simulink model "inv_rot_pen_sldrt_uart_com"  (R2024a)
settings: Solver=ode3  StartTime=0.0  StopTime=inf  FixedStep=Ts  RelTol=1e-3
PostLoadFcn:
  | try
  | if isempty(which('ZHAWcbfcn'));
  | callback_fid07124=fopen('ZHAWcbfcn.m','w');
  | [~]=fprintf(callback_fid07124,'%s',get_param([bdroot,'/ Setup SLDRT'],'ClipboardFcn'));
  | [~]=fclose(callback_fid07124);
  | setpref('ZHAW_SLDRT_lib','cb_fcn',which('ZHAWcbfcn'))
  | clear callback_fid07124
  | end
  | catch
  | clear callback_fid07124
  | end
  | Ts=eval(get_param([bdroot,'/ Setup SLDRT'],'Ts'));
InitFcn:
  | Ts=eval(get_param([bdroot,'/ Setup SLDRT'],'Ts'));
values from neighbouring files (symbols this model uses):
  i_max = 0.5    [inv_rot_pen_ini.m]    (also in swing_up_inv_rot_pen_ini.m)
  phi2_disable = 10 * pi/180    (= 0.174532925199)    [inv_rot_pen_ini.m]
  phi2_enable = 30 * pi/180    (= 0.523598775598)    [inv_rot_pen_ini.m]
  V = 1 / dc(1)    [inv_rot_pen_ini.m]
undefined symbols (not defined in the file or in its folder): K, Serial_Port, Standard_Devices
libraries: sldrtlib x3, cstblocks x2
(part 2 of 2)

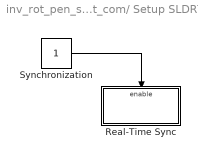
== system inv_rot_pen_sldrt_uart_com/ Setup SLDRT ==
  Real-Time Sync : Subsystem
  Synchronization : Constant
  wires:
  Synchronization/1 -> Real-Time Sync/Enable

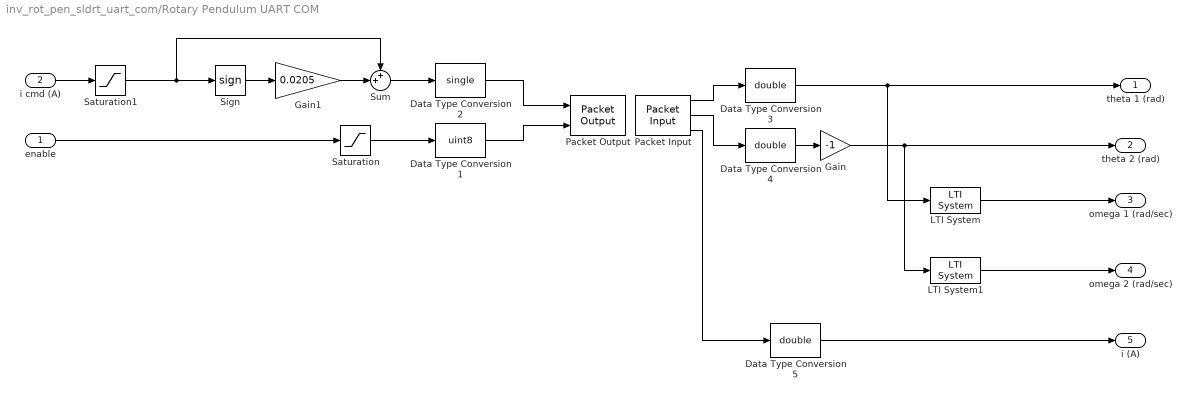
== system inv_rot_pen_sldrt_uart_com/Rotary Pendulum UART COM ==
  enable : Inport
  i cmd (A) : Inport  Port=2
  Data Type Conversion1 : DataTypeConversion  OutDataTypeStr=uint8  SaturateOnIntegerOverflow=off  RndMeth=Floor
  Data Type Conversion2 : DataTypeConversion  OutDataTypeStr=single  SaturateOnIntegerOverflow=off  RndMeth=Floor
  Data Type Conversion3 : DataTypeConversion  OutDataTypeStr=double  SaturateOnIntegerOverflow=off  RndMeth=Floor
  Data Type Conversion4 : DataTypeConversion  OutDataTypeStr=double  SaturateOnIntegerOverflow=off  RndMeth=Floor
  Data Type Conversion5 : DataTypeConversion  OutDataTypeStr=double  SaturateOnIntegerOverflow=off  RndMeth=Floor
  Gain : Gain  Gain=-1
  Gain1 : Gain  Gain=0.0205
  LTI System : cstblocks/LTI System  sys=G_diff  IC=[]  PadeOrder=0
  LTI System1 : cstblocks/LTI System  sys=G_diff  IC=[]  PadeOrder=0
  Packet Input : sldrtlib/Packet Input  SampleTime=Ts  MaxMissedTicks=10  ShowMissedTicks=off  YieldWhenWaiting=off  DrvName=Standard_Devices/Serial_Port  DrvAddress=8  DrvOptions=[115200 8 0 0 0 0 0 0]  PacketSize=4 + 4 + 4  DataTypes={'single', 'single', 'single'}  ShowReady=off  ShowError=off  PacketID=1  ByteOrder=1  ShowTimestamp=off
      settings: AttributesFormatString=Serial Port [8]
  Packet Output : sldrtlib/Packet Output  SampleTime=Ts  MaxMissedTicks=10  ShowMissedTicks=off  YieldWhenWaiting=off  DrvName=Standard_Devices/Serial_Port  DrvAddress=8  DrvOptions=[115200 8 0 0 0 0 0 0]  PacketSize=4 + 1  DataTypes={'single', 'uint8'}  ShowReady=off  ShowError=off  PacketID=1  ByteOrder=1  InitialValue=[]  FinalValue=[]
      settings: AttributesFormatString=Serial Port [8]
  Saturation : Saturate  UpperLimit=1.0  LowerLimit=0.0
  Saturation1 : Saturate  UpperLimit=i_max  LowerLimit=-i_max
  Sign : Signum
  Sum : Sum  Inputs=++|
  theta 1 (rad) : Outport
  theta 2 (rad) : Outport  Port=2
  omega 1 (rad/sec) : Outport  Port=3
  omega 2 (rad/sec) : Outport  Port=4
  i (A) : Outport  Port=5
  wires:
  Data Type Conversion2/1 -> Packet Output/1
  Packet Input/2 -> Data Type Conversion4/1
  Saturation/1 -> Data Type Conversion1/1
  Packet Input/1 -> Data Type Conversion3/1
  Data Type Conversion1/1 -> Packet Output/2
  enable/1 -> Saturation/1
  Data Type Conversion3/1 -> LTI System/1, theta 1 (rad)/1
  Data Type Conversion4/1 -> Gain/1
  LTI System/1 -> omega 1 (rad/sec)/1
  LTI System1/1 -> omega 2 (rad/sec)/1
  Gain/1 -> LTI System1/1, theta 2 (rad)/1
  Packet Input/3 -> Data Type Conversion5/1
  Data Type Conversion5/1 -> i (A)/1
  Sign/1 -> Gain1/1
  Gain1/1 -> Sum/2
  i cmd (A)/1 -> Saturation1/1
  Sum/1 -> Data Type Conversion2/1
  Saturation1/1 -> Sum/1, Sign/1

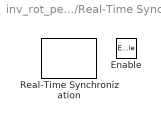
== system inv_rot_pen_sldrt_uart_com/ Setup SLDRT/Real-Time Sync ==
  Enable : EnablePort
  Real-Time Synchronization : sldrtlib/Real-Time Synchronization  SampleTime=Ts  MaxMissedTicks=inf  ShowMissedTicks=off  YieldWhenWaiting=off

== matlab function inv_rot_pen_sldrt_uart_com/Enable in Bounds Once ==
  settings: updateMethod=DISCRETE  sampleTime=Ts
  data: phi2 input; Enable output; phi2_enable parameter; phi2_disable parameter
function Enable = fcn(phi2, phi2_enable, phi2_disable)
% One-shot hysteresis switch:
%  - Activates when   |phi2| <= phi2_enable   (only if never activated before)
%  - Deactivates when |phi2| >= phi2_disable  (after activation)
%  - Cannot be activated again once deactivated
%
% Inputs:
%   phi2         current angle in radians
%   phi2_enable  activation threshold (inner) in radians
%   phi2_disable deactivation threshold (outer) in radians
%
% Output:
%   Enable = 1 when active, 0 when inactive (locked after first deactivate)

    persistent active_state has_been_enabled_once
    if isempty(active_state)
        active_state = false;
        has_been_enabled_once = false;
    end

    % Normalize thresholds: ensure inner <= outer (bulletproofing #1)
    if phi2_disable < phi2_enable
        tmp = phi2_enable;
        phi2_enable = phi2_disable;
        phi2_disable = tmp;
    end

    if ~has_been_enabled_once
        % Enable once when inside the inner band (bulletproofing #2: inclusive)
        if abs(phi2) <= phi2_enable
            active_state = true;

        % After activation, disable once when outside the outer band (inclusive)
        elseif active_state && abs(phi2) >= phi2_disable
            active_state = false;
            has_been_enabled_once = true;   % lock out reactivation
        end
    end

    Enable = double(active_state);
end
